simulink model "gain_amplifier"  (R2021a)
settings: Solver=VariableStepAuto  StartTime=0.0  StopTime=1.0  RelTol=1e-3
settings Model: Creator=Acer  LastModifiedBy=Acer

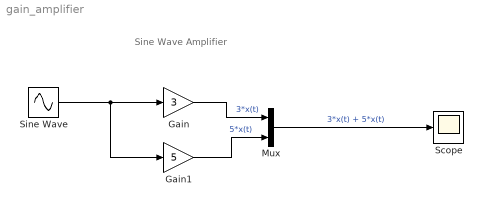
== system gain_amplifier ==
  note: Sine Wave Amplifier
  Gain : Gain  Gain=3
  Gain1 : Gain  Gain=5
  Mux : Mux  Inputs=2
  Scope : Scope
  Sine Wave : Sin  Frequency=2*pi*1  SampleTime=0
  wires:
  Sine Wave/1 -> Gain1/1, Gain/1
  Gain/1 -> Mux/1  "3*x(t)"
  Gain1/1 -> Mux/2  "5*x(t)"
  Mux/1 -> Scope/1  "3*x(t) + 5*x(t)"
